simulink model "MyTry"  (R2023b)
settings: Solver=FixedStepAuto  StartTime=0.0  StopTime=20  FixedStep=0.0005  MaxStep=0.01  RelTol=1e-3
undefined symbols (not defined in the file): centers, W
settings Model: Creator=Arshia  LastModifiedBy=ArshiaGosh

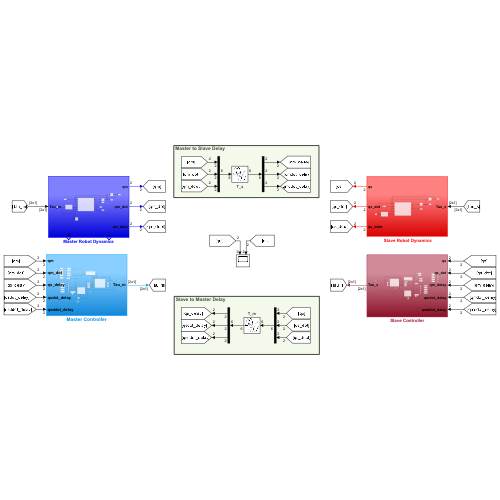
[thumbnail: Simulink's stored preview of the top-level diagram]
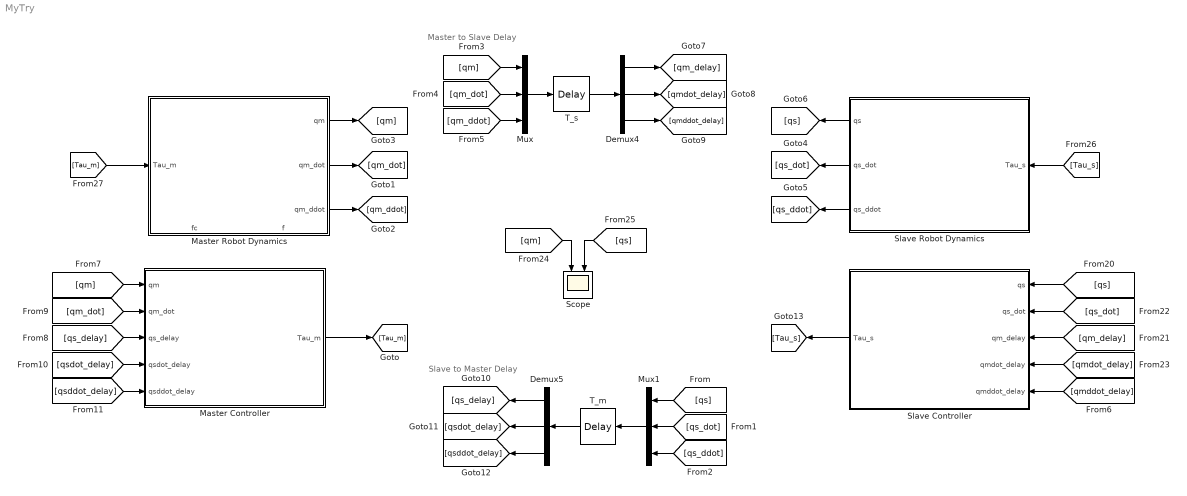
== system MyTry ==
  note: Master to Slave Delay
  note: Slave to Master Delay
  " Slave Robot Dynamics" : Subsystem
  Demux4 : Demux  Outputs=3
  Demux5 : Demux  Outputs=3
  Master Controller : Subsystem
  Master Robot Dynamics : Subsystem
      settings: PortSchema="{\"entries\":[{\"content\":{\"sides\":[{\"content\":{\"connectorIds\":[\"In1\"]},\"type\":\"ConnectorPlacement.EquallySpacedRectSide\",\"uuid\":\"608bae98-23cd-4f79-989a-683d404f42bb\"},{\"content\":{\"connectorIds\":[\"Out1\",\"Out2\",\"Out3\"],\"side\":\"RIGHT\"},\"type\":\"ConnectorPlacement.EquallySpacedRectSide\",\"uuid\":\"1c862a9e-5e7a-4999-a8d1-50cef8da0ad1\"},{\"content\":{\"side\":\"TOP\"},\"type\":\"ConnectorPlacement.EquallySpacedRectSide\",\"uuid\":\"aa4a4d3c-aa06-484c-86cd-ff210156f7cb\"},{\"content\":{\"connectorIds\":[\"Out4\",\"Out5\"],\"side\":\"BOTTOM\"},\"type\":\"ConnectorPlacement.EquallySpacedRectSide\",\"uuid\":\"07de75a6-cd81-4ece-b491-32398098d02f\"}]},\"type\":\"ConnectorPlacement.EquallySpacedConnector\",\"uuid\":\"9a93752f-4586-4942-a85a-61ba13339120\"}],\"packageUris\":[\"http://schema.mathworks.com/mf0/Connector/R2020b\"],\"version\":\"1.0\"}"
  Mux : Mux  Inputs=3
  Mux1 : Mux  Inputs=3
  Scope : Scope  NumInputPorts=2
  Slave Controller : Subsystem
      settings: PortSchema="{\"entries\":[{\"content\":{\"sides\":[{\"content\":{\"connectorIds\":[\"Out1\"]},\"type\":\"ConnectorPlacement.EquallySpacedRectSide\",\"uuid\":\"d4a5ddb8-0a78-4a6a-b69d-d0fbf887851f\"},{\"content\":{\"connectorIds\":[\"In1\",\"In2\",\"In3\",\"In4\",\"In5\"],\"side\":\"RIGHT\"},\"type\":\"ConnectorPlacement.EquallySpacedRectSide\",\"uuid\":\"c5c29000-cc93-4062-8d85-ef113d846d4c\"},{\"content\":{\"side\":\"TOP\"},\"type\":\"ConnectorPlacement.EquallySpacedRectSide\",\"uuid\":\"9fcdc3c0-dbe1-4ddf-bcf2-0add46548f02\"}]},\"type\":\"ConnectorPlacement.EquallySpacedConnector\",\"uuid\":\"1cc86ea2-f14f-4381-9537-68d258fe8551\"}],\"packageUris\":[\"http://schema.mathworks.com/mf0/Connector/R2020b\"],\"version\":\"1.0\"}"
  T_m : TransportDelay  DelayTime=0.001  BufferSize=1024*1024
  T_s : TransportDelay  DelayTime=0.001  BufferSize=1024*1024
  wires:
  Mux/1 -> T_s/1
  Mux1/1 -> T_m/1
  Master Robot Dynamics/1(qm) -> [qm]
  Master Robot Dynamics/2(qm_dot) -> [qm_dot]
  Master Robot Dynamics/3(qm_ddot) -> [qm_ddot]
  " Slave Robot Dynamics"/1(qs) -> [qs]
  " Slave Robot Dynamics"/3(qs_ddot) -> [qs_ddot]
  " Slave Robot Dynamics"/2(qs_dot) -> [qs_dot]
  [qs] -> Mux1/1
  [qs_dot] -> Mux1/2
  [qs_ddot] -> Mux1/3
  [qm] -> Mux/1
  [qm_dot] -> Mux/2
  [qm_ddot] -> Mux/3
  T_s/1 -> Demux4/1
  Demux4/1 -> [qm_delay]
  Demux4/2 -> [qmdot_delay]
  Demux4/3 -> [qmddot_delay]
  Demux5/1 -> [qs_delay]
  T_m/1 -> Demux5/1
  Demux5/3 -> [qsddot_delay]
  Demux5/2 -> [qsdot_delay]
  [qm] -> Scope/1
  [qs] -> Scope/2
  [Tau_s] -> " Slave Robot Dynamics"/1(Tau_s)
  [Tau_m] -> Master Robot Dynamics/1(Tau_m)
  Master Controller/1(Tau_m) -> [Tau_m]
  Slave Controller/1(Tau_s) -> [Tau_s]
  [qs] -> Slave Controller/1(qs)
  [qm_delay] -> Slave Controller/3(qm_delay)
  [qs_dot] -> Slave Controller/2(qs_dot)
  [qmdot_delay] -> Slave Controller/4(qmdot_delay)
  [qmddot_delay] -> Slave Controller/5(qmddot_delay)
  [qm] -> Master Controller/1(qm)
  [qm_dot] -> Master Controller/2(qm_dot)
  [qs_delay] -> Master Controller/3(qs_delay)
  [qsdot_delay] -> Master Controller/4(qsdot_delay)
  [qsddot_delay] -> Master Controller/5(qsddot_delay)

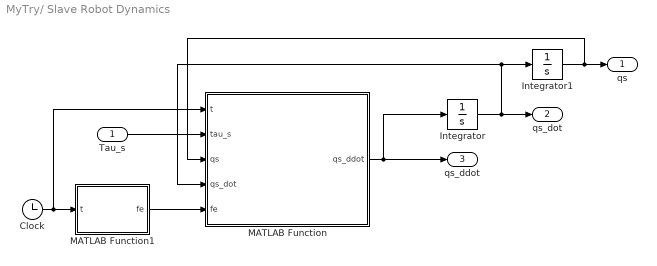
== system MyTry/ Slave Robot Dynamics ==
  Tau_s : Inport
  Clock : Clock
  Integrator : Integrator  InitialCondition=[0;0]
  Integrator1 : Integrator  InitialCondition=[0.25*pi; 0.1*pi]
  MATLAB Function : MATLAB Function  TreatAsAtomicUnit=on
  MATLAB Function1 : MATLAB Function  TreatAsAtomicUnit=on
  qs : Outport
  qs_dot : Outport  Port=2
  qs_ddot : Outport  Port=3
  wires:
  Clock/1 -> MATLAB Function/1(t), MATLAB Function1/1(t)
  Integrator1/1 -> MATLAB Function/3(qs), qs/1
  Integrator/1 -> MATLAB Function/4(qs_dot), Integrator1/1, qs_dot/1
  MATLAB Function/1(qs_ddot) -> qs_ddot/1, Integrator/1
  Tau_s/1 -> MATLAB Function/2(tau_s)
  MATLAB Function1/1(fe) -> MATLAB Function/5(fe)

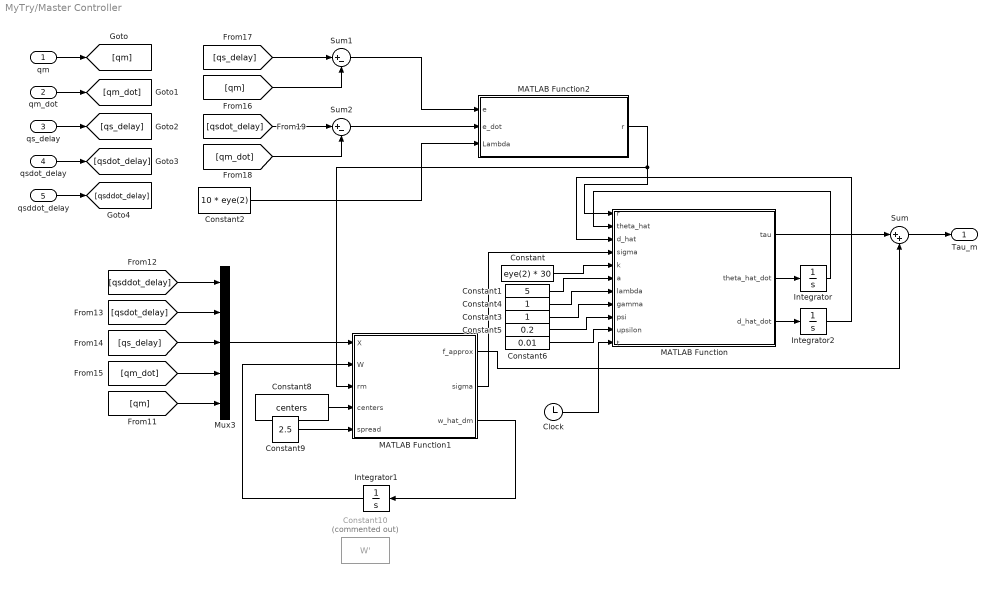
== system MyTry/Master Controller ==
  qm : Inport
  qm_dot : Inport  Port=2
  qs_delay : Inport  Port=3
  qsdot_delay : Inport  Port=4
  qsddot_delay : Inport  Port=5
  Clock : Clock
  Constant : Constant  Value=eye(2) * 30
  Constant1 : Constant  Value=5
  Constant10 : Constant  Commented=on  Value=W'
  Constant2 : Constant  Value=10 * eye(2)
  Constant3 : Constant
  Constant4 : Constant
  Constant5 : Constant  Value=0.2
  Constant6 : Constant  Value=0.01
  Constant8 : Constant  Value=centers
  Constant9 : Constant  Value=2.5
  Integrator : Integrator
  Integrator1 : Integrator  InitialCondition=W' .* eye(10,2)
  Integrator2 : Integrator
  MATLAB Function : MATLAB Function  TreatAsAtomicUnit=on
  MATLAB Function1 : MATLAB Function  TreatAsAtomicUnit=on
  MATLAB Function2 : MATLAB Function  TreatAsAtomicUnit=on
  Mux3 : Mux  Inputs=5
  Sum : Sum  Inputs=|++
  Sum1 : Sum  Inputs=|+-
  Sum2 : Sum  Inputs=|+-
  Tau_m : Outport
  wires:
  Integrator1/1 -> MATLAB Function1/2(W)
  Constant4/1 -> MATLAB Function/7(lambda)
  MATLAB Function/1(tau) -> Sum/1
  Constant1/1 -> MATLAB Function/6(a)
  Integrator2/1 -> MATLAB Function/3(d_hat)
  Constant8/1 -> MATLAB Function1/4(centers)
  [qm] -> Sum1/2
  MATLAB Function/2(theta_hat_dot) -> Integrator/1
  [qm_dot] -> Mux3/4
  MATLAB Function/3(d_hat_dot) -> Integrator2/1
  MATLAB Function2/1(r) -> MATLAB Function1/3(rm), MATLAB Function/1(r)
  Constant2/1 -> MATLAB Function2/3(Lambda)
  Constant6/1 -> MATLAB Function/10(upsilon)
  Constant5/1 -> MATLAB Function/9(psi)
  Mux3/1 -> MATLAB Function1/1(X)
  MATLAB Function1/2(sigma) -> MATLAB Function/4(sigma)
  Constant9/1 -> MATLAB Function1/5(spread)
  [qsddot_delay] -> Mux3/1
  [qsdot_delay] -> Sum2/1
  Constant/1 -> MATLAB Function/5(k)
  Integrator/1 -> MATLAB Function/2(theta_hat)
  Clock/1 -> MATLAB Function/11(t)
  Constant3/1 -> MATLAB Function/8(gamma)
  Sum/1 -> Tau_m/1
  [qm_dot] -> Sum2/2
  [qm] -> Mux3/5
  Sum1/1 -> MATLAB Function2/1(e)
  [qs_delay] -> Sum1/1
  [qs_delay] -> Mux3/3
  [qsdot_delay] -> Mux3/2
  qs_delay/1 -> [qs_delay]
  qm/1 -> [qm]
  qm_dot/1 -> [qm_dot]
  qsdot_delay/1 -> [qsdot_delay]
  qsddot_delay/1 -> [qsddot_delay]
  Sum2/1 -> MATLAB Function2/2(e_dot)
  MATLAB Function1/1(f_approx) -> Sum/2
  MATLAB Function1/3(w_hat_dm) -> Integrator1/1

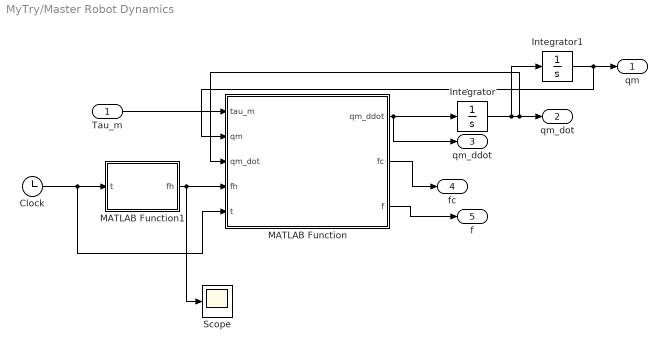
== system MyTry/Master Robot Dynamics ==
  Tau_m : Inport
  Clock : Clock
  Integrator : Integrator  InitialCondition=[0;0]
  Integrator1 : Integrator  InitialCondition=[0.4*pi; 0.2*pi]
  MATLAB Function : MATLAB Function  TreatAsAtomicUnit=on
  MATLAB Function1 : MATLAB Function  TreatAsAtomicUnit=on
  Scope : Scope
  qm : Outport
  qm_dot : Outport  Port=2
  qm_ddot : Outport  Port=3
  fc : Outport  Port=4
  f : Outport  Port=5
  wires:
  MATLAB Function/1(qm_ddot) -> qm_ddot/1, Integrator/1
  Integrator/1 -> Integrator1/1, MATLAB Function/3(qm_dot), qm_dot/1
  Integrator1/1 -> MATLAB Function/2(qm), qm/1
  Tau_m/1 -> MATLAB Function/1(tau_m)
  MATLAB Function1/1(fh) -> Scope/1, MATLAB Function/4(fh)
  Clock/1 -> MATLAB Function1/1(t), MATLAB Function/5(t)
  MATLAB Function/2(fc) -> fc/1
  MATLAB Function/3(f) -> f/1

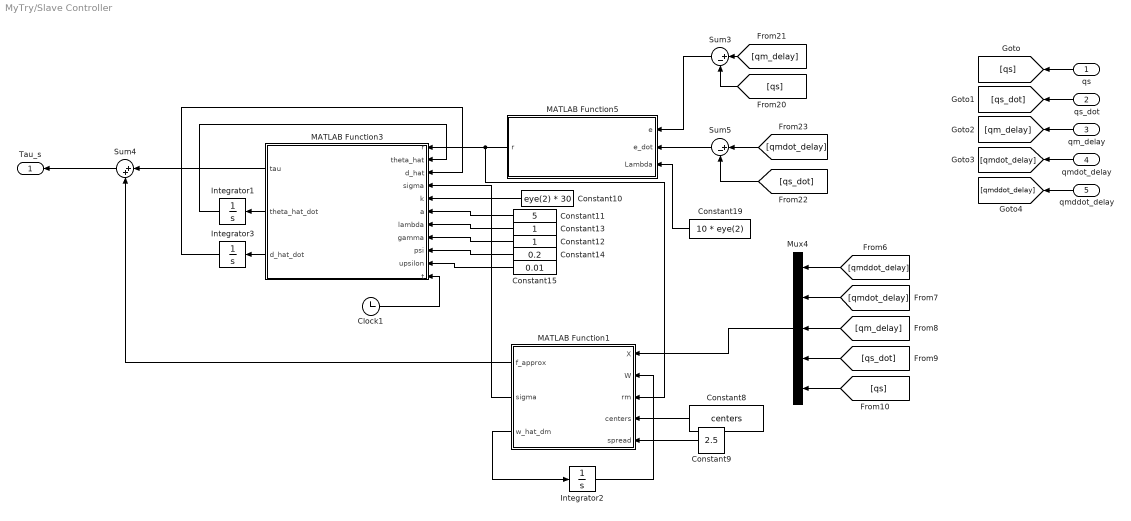
== system MyTry/Slave Controller ==
  qs : Inport
  qs_dot : Inport  Port=2
  qm_delay : Inport  Port=3
  qmdot_delay : Inport  Port=4
  qmddot_delay : Inport  Port=5
  Clock1 : Clock
  Constant10 : Constant  Value=eye(2) * 30
  Constant11 : Constant  Value=5
  Constant12 : Constant
  Constant13 : Constant
  Constant14 : Constant  Value=0.2
  Constant15 : Constant  Value=0.01
  Constant19 : Constant  Value=10 * eye(2)
  Constant8 : Constant  Value=centers
  Constant9 : Constant  Value=2.5
  Integrator1 : Integrator
  Integrator2 : Integrator  InitialCondition=W' .* eye(10,2)
  Integrator3 : Integrator
  MATLAB Function1 : MATLAB Function  TreatAsAtomicUnit=on
  MATLAB Function3 : MATLAB Function  TreatAsAtomicUnit=on
  MATLAB Function5 : MATLAB Function  TreatAsAtomicUnit=on
  Mux4 : Mux  Inputs=5
  Sum3 : Sum  Inputs=|+-
  Sum4 : Sum  Inputs=|++
  Sum5 : Sum  Inputs=|+-
  Tau_s : Outport
  wires:
  [qs] -> Mux4/5
  Constant12/1 -> MATLAB Function3/8(gamma)
  Sum4/1 -> Tau_s/1
  Constant13/1 -> MATLAB Function3/7(lambda)
  MATLAB Function3/1(tau) -> Sum4/1
  Constant15/1 -> MATLAB Function3/10(upsilon)
  Integrator3/1 -> MATLAB Function3/3(d_hat)
  Constant14/1 -> MATLAB Function3/9(psi)
  Constant19/1 -> MATLAB Function5/3(Lambda)
  Sum3/1 -> MATLAB Function5/1(e)
  Integrator1/1 -> MATLAB Function3/2(theta_hat)
  Constant11/1 -> MATLAB Function3/6(a)
  [qmdot_delay] -> Sum5/1
  Clock1/1 -> MATLAB Function3/11(t)
  [qmdot_delay] -> Mux4/2
  MATLAB Function3/2(theta_hat_dot) -> Integrator1/1
  [qmddot_delay] -> Mux4/1
  Constant10/1 -> MATLAB Function3/5(k)
  MATLAB Function3/3(d_hat_dot) -> Integrator3/1
  [qm_delay] -> Sum3/1
  [qm_delay] -> Mux4/3
  [qs] -> Sum3/2
  [qs_dot] -> Mux4/4
  [qs_dot] -> Sum5/2
  qs/1 -> [qs]
  qs_dot/1 -> [qs_dot]
  qm_delay/1 -> [qm_delay]
  qmdot_delay/1 -> [qmdot_delay]
  qmddot_delay/1 -> [qmddot_delay]
  Sum5/1 -> MATLAB Function5/2(e_dot)
  MATLAB Function1/3(w_hat_dm) -> Integrator2/1
  Constant8/1 -> MATLAB Function1/4(centers)
  MATLAB Function1/2(sigma) -> MATLAB Function3/4(sigma)
  Integrator2/1 -> MATLAB Function1/2(W)
  MATLAB Function5/1(r) -> MATLAB Function1/3(rm), MATLAB Function3/1(r)
  Constant9/1 -> MATLAB Function1/5(spread)
  Mux4/1 -> MATLAB Function1/1(X)
  MATLAB Function1/1(f_approx) -> Sum4/2

== matlab function MyTry/Slave Controller/MATLAB Function1 ==
  data: X input; f_approx output; W input; rm input; centers input; spread input; sigma output; w_hat_dm output
function [f_approx, sigma, w_hat_dm]  = rbf_network(X, W, rm, centers, spread)
    % X: input vector [q_ddot, q_dot, q, delayed_signals]
    % Gaussian basis functions
    sigma = zeros(length(centers), 1);
    for i = 1:length(centers)
        sigma(i) = exp(-norm(X - centers(i,:))^2 / spread^2);
    end
    f_approx = W' * sigma;
    Qm=1*eye(10);
    Bm=0.5*eye(10);
    w_hat_dm=-(pinv(Qm))'*sigma*rm'-(pinv(Qm))'*Bm*W;
end

== matlab function MyTry/Slave Controller/MATLAB Function5 ==
  data: e input; r output; e_dot input; Lambda input
function r  = sliding_mode(e, e_dot, Lambda)
    r = e_dot + Lambda * e;
end

== matlab function MyTry/Master Robot Dynamics/MATLAB Function1 ==
  data: t input; fh output
function fh  = operator_force(t)
   fh = [25*(0 - cos(pi*t)); 0]; % From paper
   %fh = [25; 0]; % From paper

   % fh = [25; 0]; % From paper

end

== matlab function MyTry/Master Robot Dynamics/MATLAB Function ==
  data: tau_m input; qm_ddot output size=2; qm input; qm_dot input size=2; fh input; t input; fc output; f output
function [qm_ddot, fc, f]  = master_dynamics(tau_m, qm, qm_dot, fh, t)
    % Robot parameters from Table 2
    mm1 = 0.5; lm1 = 0.6; mm2 = 0.5; lm2 = 0.4;
    g = 9.81;
    
    % Inertia matrix
    M11 = mm1*lm1^2 + mm2*lm1^2 + mm2*lm2^2 + 2*mm2*lm1*lm2*cos(qm(2));
    M12 = mm2*lm2^2 + mm2*lm1*lm2*cos(qm(2));
    M21 = M12;
    M22 = mm2*lm2^2;
    M = [M11 M12; M21 M22];
    
    % Coriolis matrix
    C11 = -mm2*lm1*lm2*qm_dot(2)*sin(qm(2));
    C12 = -mm2*lm1*lm2*(qm_dot(1) + qm_dot(2))*sin(qm(2));
    C21 = mm2*lm1*lm2*qm_dot(1)*sin(qm(2));
    C22 = 0;
    C = [C11 C12; C21 C22];
    
    % Gravity vector
    G1 = (mm1*lm1 + mm2*lm1)*g*cos(qm(1)) + mm2*lm2*g*cos(qm(1) + qm(2));
    G2 = mm2*lm2*g*cos(qm(1) + qm(2));
    G = [G1; G2];
    
    % External disturbance
    f = [0.1*qm(1)*qm_dot(1)*sin(t); 0.1*qm(2)*qm_dot(2)*sin(t)];
    
    % Internal friction
    fc = [qm_dot(1) + 3*sign(qm_dot(1)); 2*qm_dot(2) + 2*sign(qm_dot(2))];
    
    % Solve for acceleration
    qm_ddot = M\(tau_m + fh - C*qm_dot - G - f - fc);
end

== matlab function MyTry/ Slave Robot Dynamics/MATLAB Function ==
  data: t input; qs_ddot output size=2; tau_s input; qs input; qs_dot input size=2; fe input
function qs_ddot  = slave_dynamics(t, tau_s, qs, qs_dot, fe)
    % Parameters for slave robot, from Table 2
    ms1 = 0.5; ls1 = 0.6;
    ms2 = 0.5; ls2 = 0.4;
    g = 9.81;
    
    % Inertia matrix Ms(qs)
    M11 = ms1*ls1^2 + ms2*ls1^2 + ms2*ls2^2 + 2*ms2*ls1*ls2*cos(qs(2));
    M12 = ms2*ls2^2 + ms2*ls1*ls2*cos(qs(2));
    M21 = M12;
    M22 = ms2*ls2^2;
    Ms = [M11 M12; M21 M22];
    
    % Coriolis matrix Cs(qs, qs_dot)
    C11 = -ms2*ls1*ls2*qs_dot(2)*sin(qs(2));
    C12 = -ms2*ls1*ls2*(qs_dot(1) + qs_dot(2))*sin(qs(2));
    C21 = ms2*ls1*ls2*qs_dot(1)*sin(qs(2));
    C22 = 0;
    Cs = [C11 C12; C21 C22];
    
    % Gravity vector Gs(qs)
    G1 = (ms1*ls1 + ms2*ls1)*g*cos(qs(1)) + ms2*ls2*g*cos(qs(1) + qs(2));
    G2 = ms2*ls2*g*cos(qs(1) + qs(2));
    Gs = [G1; G2];
    
    % External disturbance
    fs = [0.1*qs(1)*qs_dot(1)*sin(t); 0.1*qs(2)*qs_dot(2)*sin(t)];
    
    % Internal friction
    fc = [2*qs_dot(1) + 4*sign(qs_dot(1)); 1*qs_dot(2) + 3*sign(qs_dot(2))];
    
    % Calculate acceleration
    qs_ddot = Ms \ (tau_s + fe - Cs*qs_dot - Gs - fs - fc);
end

== matlab function MyTry/ Slave Robot Dynamics/MATLAB Function1 ==
  data: t input; fe output
function fe  = environment_force(t)
    fe = [0; 0];
end

== matlab function MyTry/Master Controller/MATLAB Function ==
  data: r input; tau output; theta_hat input; d_hat input; sigma input; k input; a input; lambda input; gamma input; psi input; upsilon input; theta_hat_dot output; d_hat_dot output; t input
function [tau, theta_hat_dot, d_hat_dot] = adaptive_controller(r, theta_hat, d_hat, sigma, k, a, lambda, gamma, psi, upsilon,t)
    % Control law (Equation 41)
    tau = k * r + (r / (2 * a^2)) * theta_hat * (sigma' * sigma) + (r / (norm(r) + exp(-a*t))) * d_hat;
%    tau = k * r + (r / (norm(r) + eps)) .* f_approx + (r / (norm(r) + exp(-a*t))) .* d_hat;

    
    % Adaptive laws (Equations 44-45)
    theta_hat_dot = (lambda / (2 * a^2)) * (r' * r) * (sigma' * sigma) - psi * theta_hat;
    d_hat_dot = (gamma * (r' * r)) / (norm(r) + exp(-a*t)) - upsilon * d_hat;
end

== matlab function MyTry/Master Controller/MATLAB Function1 ==
  data: X input; f_approx output; W input; rm input; centers input; spread input; sigma output; w_hat_dm output
function [f_approx, sigma, w_hat_dm]  = rbf_network(X, W, rm, centers, spread)
    % X: input vector [q_ddot, q_dot, q, delayed_signals]
    % Gaussian basis functions
    sigma = zeros(length(centers), 1);
    for i = 1:length(centers)
        sigma(i) = exp(-norm(X - centers(i,:))^2 / spread^2);
    end
    f_approx = W' * sigma;
    Qm=1*eye(10);
    Bm=0.5*eye(10);
    w_hat_dm=-(pinv(Qm))'*sigma*rm'-(pinv(Qm))'*Bm*W;
end

== matlab function MyTry/Master Controller/MATLAB Function2 ==
  data: e input; r output; e_dot input; Lambda input
function r  = sliding_mode(e, e_dot, Lambda)
    r = e_dot + Lambda * e;
end

== matlab function MyTry/Slave Controller/MATLAB Function3 ==
  data: r input; tau output; theta_hat input; d_hat input; sigma input; k input; a input; lambda input; gamma input; psi input; upsilon input; theta_hat_dot output; d_hat_dot output; t input
function [tau, theta_hat_dot, d_hat_dot] = adaptive_controller(r, theta_hat, d_hat, sigma, k, a, lambda, gamma, psi, upsilon, t)
    % Control law (Equation 41)
    tau = k * r + (r / (2 * a^2)) * theta_hat * (sigma' * sigma) + (r / (norm(r) + exp(-a*t))) * d_hat;
    %tau = k * r + (r / (norm(r) + eps)) .* f_approx + (r / (norm(r) + exp(-a*t))) .* d_hat;

    % Adaptive laws (Equations 44-45)
    theta_hat_dot = (lambda / (2 * a^2)) * (r' * r) * (sigma' * sigma) - psi * theta_hat;
    d_hat_dot = (gamma * (r' * r)) / (norm(r) + exp(-a*t)) - upsilon * d_hat;
end
